simulink model "questao2d"  (Simulink 3.00)
settings: Solver=ode45  StartTime=0.0  StopTime=10.0  RelTol=1e-3
libraries: simulink3 x1

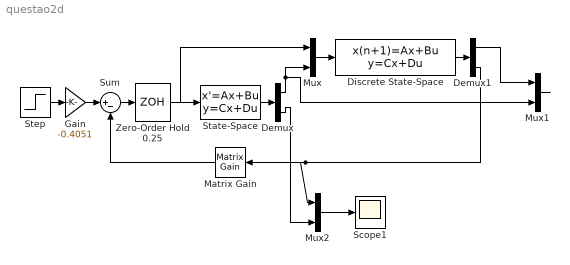
== system questao2d ==
  Demux : Demux  Outputs=2
  Demux1 : Demux  Outputs=2
  Discrete State-Space : DiscreteStateSpace  A=[-334.45830.7013 -336.8355;905.2576 6.4753 889.5;9.9555 -0.1312 12.0095]  B=[0.0045 336.9011;0.0656 -888.7331;0.2835 -107349]  C=[1 0 1;1 0 0;0 1 0;0 0 1]  D=[0 0;0 0;0 0;0 0]  X0=0  SampleTime=1
  Gain : Gain  Gain=-0.4051  SaturateOnIntegerOverflow=on
  Matrix Gain : simulink3/Math/Matrix Gain  Orientation=left  K=[229.7529 82.7326 10.3266]
  Mux : Mux  Inputs=2
  Mux1 : Mux  Inputs=2
  Mux2 : Mux  Inputs=2
  Scope1 : Scope
      settings: TimeRange=auto  YMin=-5  YMax=5  SaveToWorkspace=off  SaveName=ScopeData
  State-Space : StateSpace  A=[0 1 0 ;5.75 23.75 1; -2 0 1 ]  B=[0; 0 ;1]  C=[1 0 1;eye(3,3)]  D=[0;0;0;0]  X0=0
  Step : Step  Time=1  Before=0  After=1  SampleTime=0
  Sum : Sum  Inputs=|+-  SaturateOnIntegerOverflow=on
  Zero-Order Hold 0.25 : ZeroOrderHold  SampleTime=0.25
  wires:
  Zero-Order Hold 0.25/1 -> State-Space/1, Mux/1
  State-Space/1 -> Demux/1
  Mux/1 -> Discrete State-Space/1
  Discrete State-Space/1 -> Demux1/1
  Mux1/1 -> ?
  Demux1/1 -> Mux1/1
  Step/1 -> Gain/1
  Demux/1 -> Mux/2, Mux1/2
  Gain/1 -> Sum/1
  Sum/1 -> Zero-Order Hold 0.25/1
  Matrix Gain/1 -> Sum/2
  Mux2/1 -> Scope1/1
  Demux/2 -> Mux2/2
  Demux1/2 -> Matrix Gain/1, Mux2/1
